simulink model "cxema4"  (R2014a)
settings: Solver=ode45  StartTime=0.0  StopTime=50  MaxStep=0.001  MinStep=0.0001  RelTol=1e-3
settings Model: Creator=User  LastModifiedBy=User

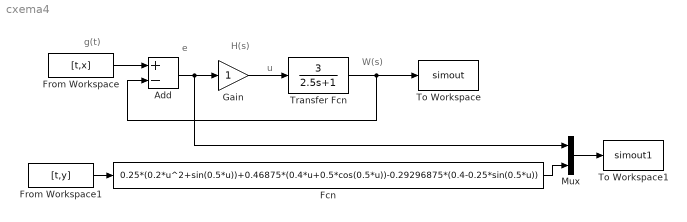
== system cxema4 ==
  note: W(s)
  note: H(s)
  note: u
  note: g(t)
  note: e
  Add : Sum  Inputs=+-
  Fcn : Fcn  Expr=0.25*(0.2*u^2+sin(0.5*u))+0.46875*(0.4*u+0.5*cos(0.5*u))-0.29296875*(0.4-0.25*sin(0.5*u))
  From Workspace : FromWorkspace  VariableName=[t,x]  SampleTime=0
  From Workspace1 : FromWorkspace  VariableName=[t,y]  SampleTime=0
  Gain : Gain
  Mux : Mux  Inputs=2
  To Workspace : ToWorkspace  VariableName=simout  SaveFormat=Timeseries  SampleTime=-1
  To Workspace1 : ToWorkspace  VariableName=simout1  SaveFormat=Timeseries  SampleTime=-1
  Transfer Fcn : TransferFcn  Numerator=[3]  Denominator=[2.5 1]
  wires:
  Gain/1 -> Transfer Fcn/1
  Add/1 -> Mux/1, Gain/1
  From Workspace/1 -> Add/1
  Transfer Fcn/1 -> Add/2, To Workspace/1
  Mux/1 -> To Workspace1/1
  From Workspace1/1 -> Fcn/1
  Fcn/1 -> Mux/2
